simulink model "projekat1zatvorenasprega"  (R2021a)
settings: Solver=ode4  StartTime=0.0  StopTime=1000000.0  FixedStep=0.1  RelTol=1e-3
values from neighbouring files (symbols this model uses):
  Ca = 10^-6    (= 1e-06)    [projekat1.m]
  Cb = 10^-6    (= 1e-06)    [projekat1.m]
  Fa = 0.016667    [projekat1.m]
  K = 10000000    [projekat1.m]
  kw = 10^-14    (= 1e-14)    [projekat1.m]
  V = 30    [projekat1.m]
settings Model: Creator=Dusan Licina  LastModifiedBy=svorc
settings SolverCC: AlgebraicLoopSolver=TrustRegion
settings DataIOCC: ReturnWorkspaceOutputs=off
settings DebuggingCC: SFMachineParentedDataDiag=warning  ArithmeticOperatorsInVariantConditions=warning
settings SFSimCC: SimUseLocalCustomCode=off  CustomCodeUndefinedFunction=UseInterfaceOnly
settings RTWCC: RTWUseLocalCustomCode=off

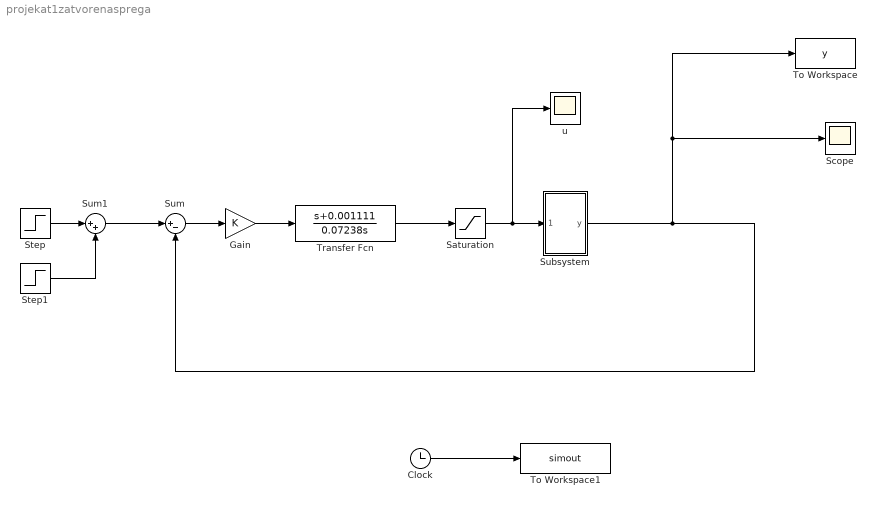
== system projekat1zatvorenasprega ==
  Clock : Clock
  Gain : Gain  Gain=K
  Saturation : Saturate  UpperLimit=10*Fa  LowerLimit=0
  Scope : Scope
  Step : Step  Time=0.1  After=7  SampleTime=0
  Step1 : Step  Time=100000  SampleTime=0
  Subsystem : Subsystem
  Sum : Sum  Inputs=|+-
  Sum1 : Sum  Inputs=|++
  To Workspace : ToWorkspace  VariableName=y  SampleTime=-1
  To Workspace1 : ToWorkspace  VariableName=simout  SampleTime=-1
  Transfer Fcn : TransferFcn  Numerator=[1 0.001111]  Denominator=[0.07238 0]
  u : Scope
  wires:
  Transfer Fcn/1 -> Saturation/1
  Step1/1 -> Sum1/2
  Step/1 -> Sum1/1
  Sum1/1 -> Sum/1
  Subsystem/1(y) -> Sum/2, Scope/1, To Workspace/1
  Saturation/1 -> u/1, Subsystem/1(Input)
  Sum/1 -> Gain/1
  Gain/1 -> Transfer Fcn/1
  Clock/1 -> To Workspace1/1

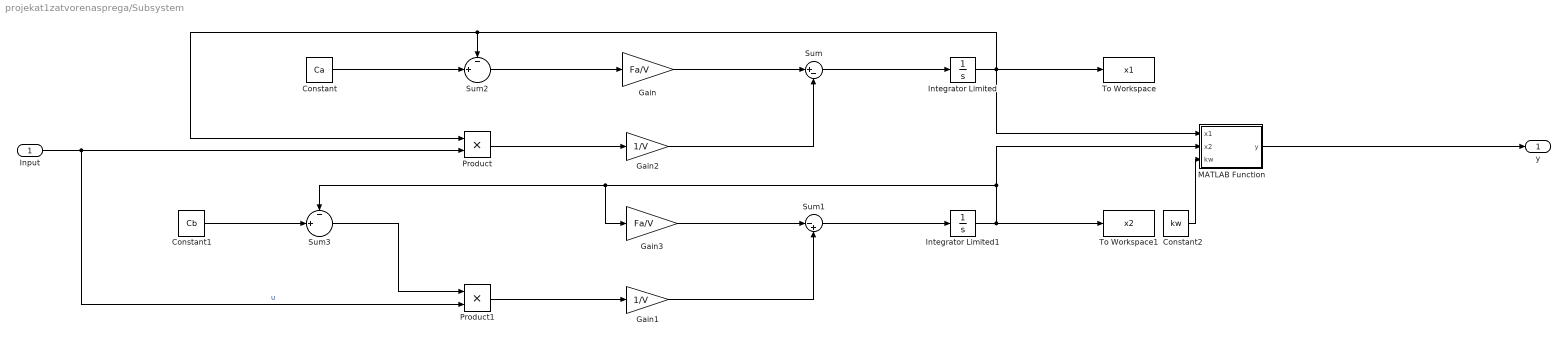
== system projekat1zatvorenasprega/Subsystem ==
  Input : Inport
  Constant : Constant  Value=Ca
  Constant1 : Constant  Value=Cb
  Constant2 : Constant  Value=kw
  Gain : Gain  Gain=Fa/V
  Gain1 : Gain  Gain=1/V
  Gain2 : Gain  Gain=1/V
  Gain3 : Gain  Gain=Fa/V
  Integrator Limited : Integrator  LimitOutput=on  UpperSaturationLimit=Ca  LowerSaturationLimit=0
  Integrator Limited1 : Integrator  LimitOutput=on  UpperSaturationLimit=Cb  LowerSaturationLimit=0
  MATLAB Function : MATLAB Function  TreatAsAtomicUnit=on
  Product : Product
  Product1 : Product
  Sum : Sum  Inputs=|+-
  Sum1 : Sum  Inputs=|-+
  Sum2 : Sum  Inputs=-|+||
  Sum3 : Sum  Inputs=-|+||
  To Workspace : ToWorkspace  VariableName=x1  SampleTime=-1
  To Workspace1 : ToWorkspace  VariableName=x2  SampleTime=-1
  y : Outport
  wires:
  Sum3/1 -> Product1/1
  Sum/1 -> Integrator Limited/1
  Gain/1 -> Sum/1
  Input/1 -> Product/2, Product1/2  "u"
  Gain3/1 -> Sum1/1
  Integrator Limited1/1 -> MATLAB Function/2(x2), Gain3/1, Sum3/1, To Workspace1/1
  Integrator Limited/1 -> To Workspace/1, MATLAB Function/1(x1), Sum2/1, Product/1
  Constant1/1 -> Sum3/2
  Sum1/1 -> Integrator Limited1/1
  Product1/1 -> Gain1/1
  Constant/1 -> Sum2/2
  Gain2/1 -> Sum/2
  MATLAB Function/1(y) -> y/1
  Gain1/1 -> Sum1/2
  Product/1 -> Gain2/1
  Sum2/1 -> Gain/1
  Constant2/1 -> MATLAB Function/3(kw)

== matlab function projekat1zatvorenasprega/Subsystem/MATLAB Function ==
  data: x1 input; y output; x2 input; kw input
function y = fcn(x1, x2, kw)

y = -log10(sqrt((x2-x1)^2 / 4 + kw) - (x2 - x1) / 2);
